simulink model "Vehicle_Dynamics_Test_Simulink"  (R2019a)
settings: Solver=FixedStepAuto  StartTime=0.0  StopTime=300  FixedStep=0.01  RelTol=1e-3
values from neighbouring files (symbols this model uses):
  Braking = Simulink.Parameter    [Vehicle_Dynamics_Script.m]
  Pedalling_Force = Simulink.Parameter    [Vehicle_Dynamics_Script.m]
  Steering_Angle = Simulink.Parameter    [Vehicle_Dynamics_Script.m]
  Terrain = Simulink.Parameter    [Vehicle_Dynamics_Script.m]
libraries: fl_lib x9, nesl_utility x6, sdl_lib x5, simulink_extras x1, vehdynlibsteering x1, autolibshared x1
settings Model: Creator=India  LastModifiedBy=India
settings OptimizationCC: DefaultParameterBehavior=Inlined  EnhancedBackFolding=on  PassReuseOutputArgsAs=Individual arguments  OptimizeBlockOrder=speed  DifferentSizesBufferReuse=on  OptimizationCustomize=off
settings DebuggingCC: ParameterTunabilityLossMsg=error
settings SFSimCC: MATLABDynamicMemAlloc=off
settings RTWCC: SystemTargetFile=ert.tlc  TemplateMakefile=ert_default_tmf  GenerateReport=on  IncludeHyperlinkInReport=on  LaunchReport=on  GenerateTraceInfo=on  GenerateTraceReport=on  GenerateTraceReportSl=on  GenerateTraceReportSf=on  GenerateTraceReportEml=on
settings CodeAppCC: ForceParamTrailComments=on  IgnoreCustomStorageClasses=off  OperatorAnnotations=on  SimulinkDataObjDesc=on  SFDataObjDesc=on  InsertBlockDesc=on
settings ERTTargetCC: TargetLangStandard=C99 (ISO)  GenerateSampleERTMain=on  InlinedParameterPlacement=NonHierarchical  ERTCustomFileTemplate=example_file_process.tlc
settings ConfigComp: DVTestSuiteOptimization=Auto  DVDetectOutOfBounds=on  DVRebuildModelRepresentation=Always

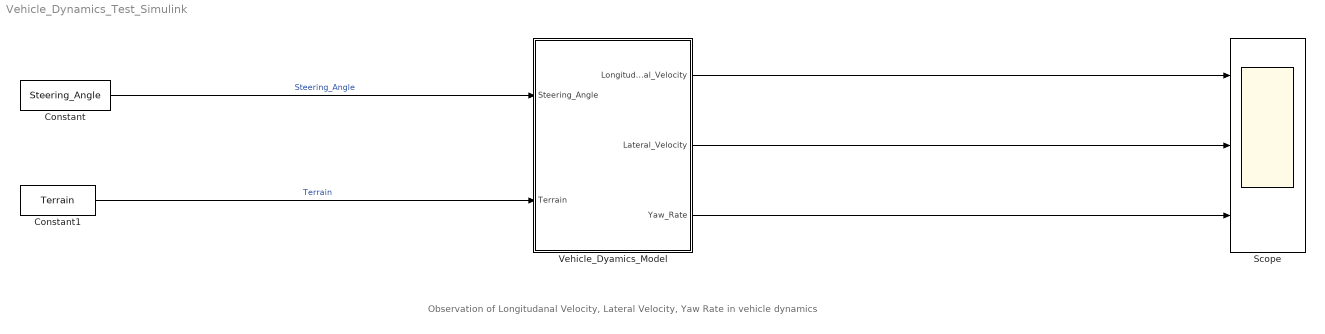
== system Vehicle_Dynamics_Test_Simulink ==
  note: Observation of Longitudanal Velocity, Lateral Velocity, Yaw Rate in vehicle dynamics
  Constant : Constant  Value=Steering_Angle  OutDataTypeStr=double
  Constant1 : Constant  Value=Terrain  OutDataTypeStr=double
  Scope : Scope  NumInputPorts=3
  Vehicle_Dyamics_Model : Subsystem  TreatAsAtomicUnit=on
  wires:
  Constant1/1 -> Vehicle_Dyamics_Model/2(Terrain)  "Terrain"
  Vehicle_Dyamics_Model/2(Lateral_Velocity) -> Scope/2
  Vehicle_Dyamics_Model/3(Yaw_Rate) -> Scope/3
  Constant/1 -> Vehicle_Dyamics_Model/1(Steering_Angle)  "Steering_Angle"
  Vehicle_Dyamics_Model/1(Longitudanal_Velocity) -> Scope/1

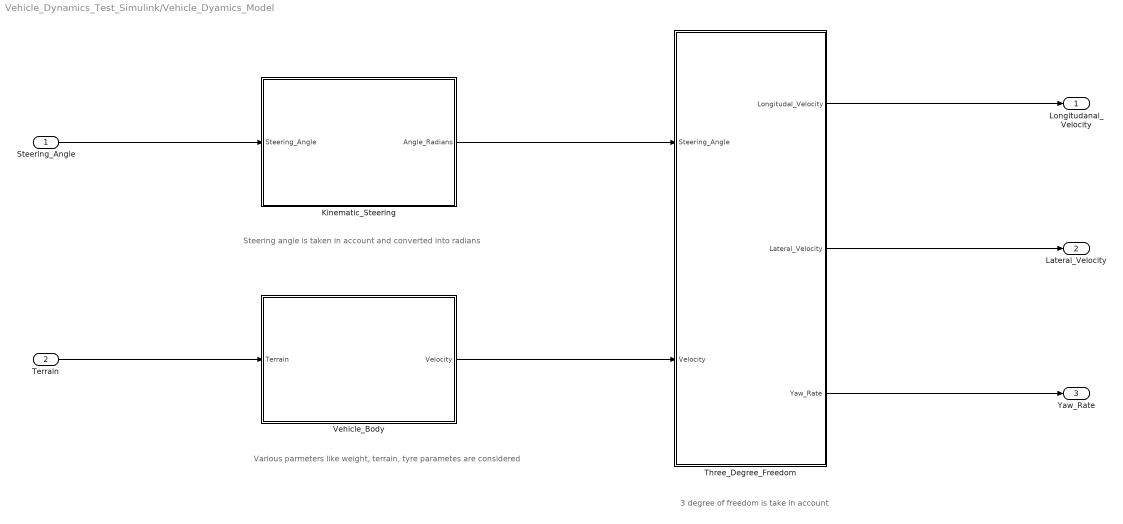
== system Vehicle_Dynamics_Test_Simulink/Vehicle_Dyamics_Model ==
  note: 3 degree of freedom is take in account
  note: Various parmeters like weight, terrain, tyre parametes are considered
  note: Steering angle is taken in account and converted into radians
  Steering_Angle : Inport
  Terrain : Inport  Port=2  OutDataTypeStr=double
  Kinematic_Steering : Subsystem
  Three_Degree_Freedom : Subsystem
  Vehicle_Body : Subsystem
  Longitudanal_Velocity : Outport
  Lateral_Velocity : Outport  Port=2
  Yaw_Rate : Outport  Port=3
  wires:
  Three_Degree_Freedom/1(Longitudal_Velocity) -> Longitudanal_Velocity/1
  Three_Degree_Freedom/2(Lateral_Velocity) -> Lateral_Velocity/1
  Vehicle_Body/1(Velocity) -> Three_Degree_Freedom/2(Velocity)
  Three_Degree_Freedom/3(Yaw_Rate) -> Yaw_Rate/1
  Kinematic_Steering/1(Angle_Radians) -> Three_Degree_Freedom/1(Steering_Angle)
  Terrain/1 -> Vehicle_Body/1(Terrain)
  Steering_Angle/1 -> Kinematic_Steering/1(Steering_Angle)

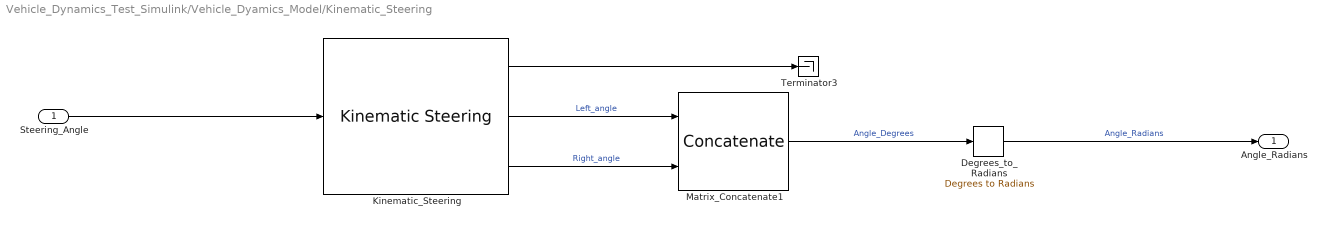
== system Vehicle_Dynamics_Test_Simulink/Vehicle_Dyamics_Model/Kinematic_Steering ==
  Steering_Angle : Inport
  Degrees_to_Radians : simulink_extras/Transformations/Degrees to Radians
  Kinematic_Steering : vehdynlibsteering/Kinematic Steering  StrgType=Ackerman  StrgRatioType=Constant  Loc=Front  NrmlFctr=0.01  TrckWdth=1  WhlBase=1.524  Db=0  StrgRng=1.25*pi  StrgAngBpts="[-6.2832   -5.0265   -3.7699   -2.5133   -1.2566         0    1.2566    2.5133    3.7699    5.0265    6.2832]"  StrgRatioTbl=|  StrgRatio=100  StrgArmLngth=0.1  RckCsLngth=0.5  TieRodLngth=0.248  D=0.2  PnnRadius=0.0057  PnnRadiusTbl="[0.0055    0.0055    0.0056    0.0057    0.0058    0.0057    0.0057    0.0057    0.0056    0.0055    0.0055]"  RodLngth=0.1  ParaArmLngth=0.9  aMode=2
      | [13.5000   13.3750   13.2500   13.1250   13.0000   13.0000   13.0000   13.1250   13.2500   13.3750   13.5000
      | ]
      settings: SourceProductName=Vehicle Dynamics Blockset
  Matrix_Concatenate1 : Concatenate  ConcatenateDimension=2
      settings: AttributesFormatString=%<ConcatenateDimension>
  Terminator3 : Terminator
  Angle_Radians : Outport
  wires:
  Kinematic_Steering/1 -> Terminator3/1
  Kinematic_Steering/3 -> Matrix_Concatenate1/2  "Right_angle"
  Matrix_Concatenate1/1 -> Degrees_to_Radians/1  "Angle_Degrees"
  Kinematic_Steering/2 -> Matrix_Concatenate1/1  "Left_angle"
  Steering_Angle/1 -> Kinematic_Steering/1
  Degrees_to_Radians/1 -> Angle_Radians/1  "Angle_Radians"

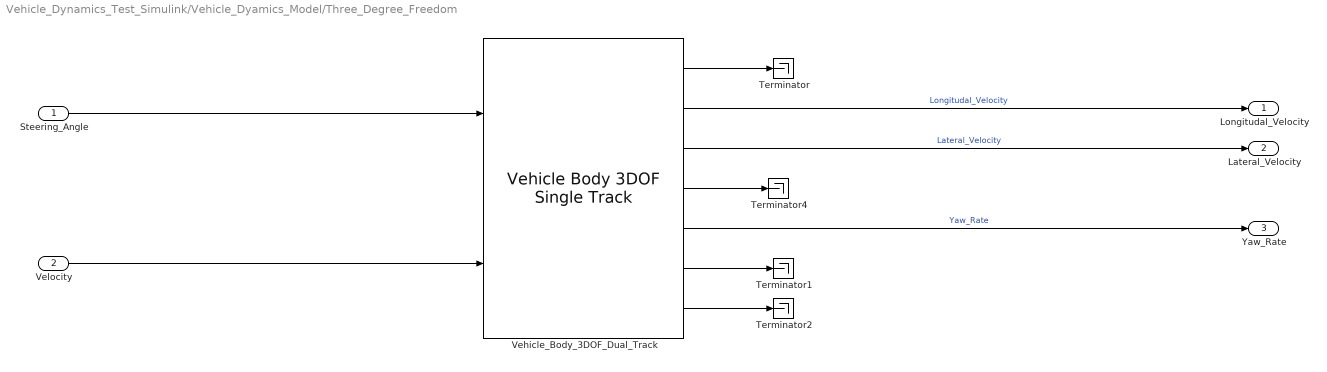
== system Vehicle_Dynamics_Test_Simulink/Vehicle_Dyamics_Model/Three_Degree_Freedom ==
  Steering_Angle : Inport
  Velocity : Inport  Port=2
  Terminator{,1..2,4} (4 alike) : Terminator
  Vehicle_Body_3DOF_Dual_Track : autolibshared/Vehicle Body 3DOF Single Track  trackMode=Dual  inputMode=External longitudinal velocity  frontSteerMode=on  rearSteerMode=off  windMode=off  muMode=off  extFMode=off  extMMode=off  extXo=off  extpsio=off  extxdoto=off  extro=off  extYo=off  extTamb=off  extydoto=off  aMode=2  NF=2  NR=2  m=2000  a=1.4  b=1.6  h=0.35  X_o=0  xdot_o=0  CalphaMode=off  sigmaMode=on  d=0  w=[1.4,1.4]  Cy_f=12e3  Cy_r=11e3  sigma_f=.1  sigma_r=.1  alpha_f_brk=[-.1 .1]  Cy_f_data=[-9e3 9e3]  alpha_r_brk=[-.1 .1]  Cy_r_data=[-9e3 9e3]  Y_o=0  ydot_o=0  Izz=4000  psi_o=0  r_o=0  Af=2  Cd=.3  Cl=.1  Cpm=.1  beta_w=[0:0.01:0.3]  Cs=[0:0.03:0.9]  Cym=[0:0.01:0.3]  Pabs=101325  Tair=273  g=9.81  mu=1  xdot_tol=.01  Fznom=5000  Fxtire_sat=7e4  Fytire_sat=7e4  longOff=0  latOff=0  vertOff=0  wrapAng=off
      settings: SourceProductName=Powertrain Blockset  SourceProductBaseCode=PW
  Longitudal_Velocity : Outport
  Lateral_Velocity : Outport  Port=2
  Yaw_Rate : Outport  Port=3
  wires:
  Vehicle_Body_3DOF_Dual_Track/3 -> Lateral_Velocity/1  "Lateral_Velocity"
  Vehicle_Body_3DOF_Dual_Track/6 -> Terminator1/1
  Velocity/1 -> Vehicle_Body_3DOF_Dual_Track/2
  Vehicle_Body_3DOF_Dual_Track/7 -> Terminator2/1
  Vehicle_Body_3DOF_Dual_Track/1 -> Terminator/1
  Vehicle_Body_3DOF_Dual_Track/4 -> Terminator4/1
  Vehicle_Body_3DOF_Dual_Track/5 -> Yaw_Rate/1  "Yaw_Rate"
  Steering_Angle/1 -> Vehicle_Body_3DOF_Dual_Track/1
  Vehicle_Body_3DOF_Dual_Track/2 -> Longitudal_Velocity/1  "Longitudal_Velocity"

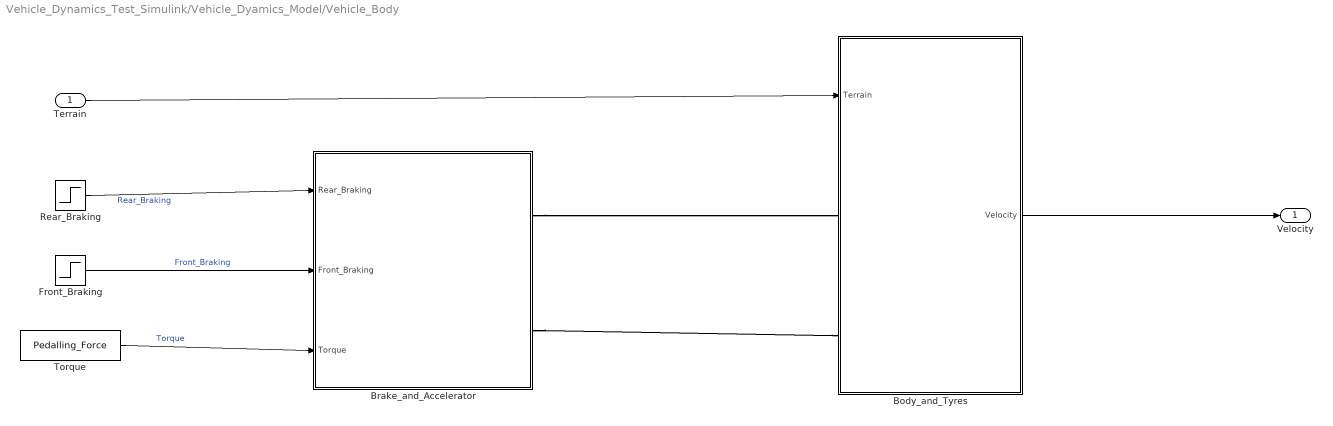
== system Vehicle_Dynamics_Test_Simulink/Vehicle_Dyamics_Model/Vehicle_Body ==
  Terrain : Inport  OutDataTypeStr=double
  Body_and_Tyres : Subsystem
  Brake_and_Accelerator : Subsystem
  Front_Braking : Step  Time=100  After=Terrain  SampleTime=0
  Rear_Braking : Step  Time=100  After=Braking  SampleTime=0
  Torque : Constant  Value=Pedalling_Force
  Velocity : Outport
  wires:
  Rear_Braking/1 -> Brake_and_Accelerator/1(Rear_Braking)  "Rear_Braking"
  Front_Braking/1 -> Brake_and_Accelerator/2(Front_Braking)  "Front_Braking"
  Torque/1 -> Brake_and_Accelerator/3(Torque)  "Torque"
  Terrain/1 -> Body_and_Tyres/1(Terrain)
  Body_and_Tyres/1(Velocity) -> Velocity/1
  connections:
  Brake_and_Accelerator/RConn1 -- Body_and_Tyres/LConn1
  Brake_and_Accelerator/RConn2 -- Body_and_Tyres/LConn2

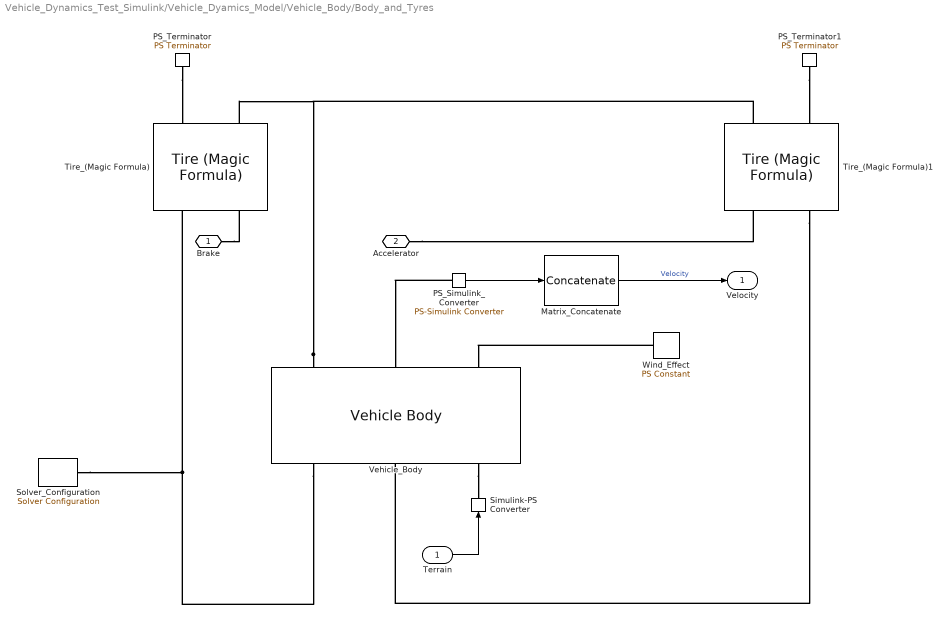
== system Vehicle_Dynamics_Test_Simulink/Vehicle_Dyamics_Model/Vehicle_Body/Body_and_Tyres ==
  Terrain : Inport
  Matrix_Concatenate : Concatenate  NumInputs=1  ConcatenateDimension=2
      settings: AttributesFormatString=%<ConcatenateDimension>
  PS_Simulink_Converter : nesl_utility/PS-Simulink Converter  PhysicalDomain=network_engine_domain  SubClassName=ps_output  LeftPortType=input  RightPortType=output  PseudoPeriodic=off  Frequencies=[]  Unit=1  AffineConversion=off
  PS_Terminator : fl_lib/Physical Signals/Sinks/PS Terminator
      settings: SourceProductName=Simscape
  PS_Terminator1 : fl_lib/Physical Signals/Sinks/PS Terminator
      settings: SourceProductName=Simscape
  Simulink-PS Converter : nesl_utility/Simulink-PS Converter  PhysicalDomain=network_engine_domain  SubClassName=ps_input  LeftPortType=input  RightPortType=output  PseudoPeriodic=off  Frequencies=[]  NoiseDistribution=none  NoiseParameters=[]  Unit=1  AffineConversion=off  FilteringAndDerivatives=provide  SimscapeFilterOrder=1  InputFilterTimeConstant=0.001  UdotUserProvided=0
  Solver_Configuration : nesl_utility/Solver Configuration  PhysicalDomain=network_engine_domain  SubClassName=solver  LeftPortType=input  RightPortType=generic  Tones=[]  Harmonics=[]  SimulateNoise=off  Profile=off  UseLocalSampling=off  EnableSwitchedLinearOptims=on  FrequencyDomain=off  UseCCode=off  RelTol=0.001  AbsTol=1e-06  MinStep=1e-09  ToWorkspace=off  RevertToSquareIcSolve=off  NumHomotopyIterations=100  PhasorMode=off  PhasorModeNumHarmonics=1  DoDC=off  ResidualTolerance=1e-09  UseLocalSolver=off  LocalSolverChoice=NE_BACKWARD_EULER_ADVANCER  LocalSolverSampleTime=0.001  DoFixedCost=off  MaxNonlinIter=3  MaxModeIter=2  LinearAlgebra=auto  EquationFormulation=NE_TIME_EF  DelaysMemoryBudget=1024  AutomaticFiltering=on  FilteringTimeConstant=0.001  PartitionStorageMethod=AS_NEEDED  PartitionMemoryBudget=1024  PartitionMethod=ROBUST
  Tire_(Magic Formula) : sdl_lib/Tires & Vehicles/Tire (Magic Formula)  parameterization=sdl.enum.magic_tire_model.constant  F_z1=3000 N  F_x1=3500 N  kappa1=10  B_m=10  C_m=1.9  D_m=1  E_m=0.97  fz0=4000 N  p_Cx=1.685  p_Dx=[1.21, -.037]  p_Ex=[.344, .095, -.02, 0]  p_Kx=[21.51, -.163, .245]  p_Hx=[-.002, .002]  p_Vx=[0, 0]  v_tr_thr=0.1 m/s  r_e=0.45 m  model_compliance=0  stiffness=1e6 N/m  damping=1000 N/(m/s)  model_inertia=1  inertia=1e-3 kg*m^2  initial_velocity=0 rad/s  model_resistance=1  resistance_model=1  coeff=0.005  p_tire=250e3 Pa  alpha=-0.003  beta=0.97  coeff_a=84e-4  coeff_b=6.2e-4 s/m  coeff_c=1.6e-4 s^2/m^2  v_thr=0.001 m/s
      settings: SourceProductName=Simscape Driveline
  Tire_(Magic Formula)1 : sdl_lib/Tires & Vehicles/Tire (Magic Formula)  parameterization=sdl.enum.magic_tire_model.constant  F_z1=3000 N  F_x1=3500 N  kappa1=10  B_m=10  C_m=1.9  D_m=1  E_m=0.97  fz0=4000 N  p_Cx=1.685  p_Dx=[1.21, -.037]  p_Ex=[.344, .095, -.02, 0]  p_Kx=[21.51, -.163, .245]  p_Hx=[-.002, .002]  p_Vx=[0, 0]  v_tr_thr=0.1 m/s  r_e=0.45 m  model_compliance=0  stiffness=1e6 N/m  damping=1000 N/(m/s)  model_inertia=1  inertia=1e-3 kg*m^2  initial_velocity=0 rad/s  model_resistance=1  resistance_model=1  coeff=0.005  p_tire=250e3 Pa  alpha=-0.003  beta=0.97  coeff_a=84e-4  coeff_b=6.2e-4 s/m  coeff_c=1.6e-4 s^2/m^2  v_thr=0.001 m/s
      settings: SourceProductName=Simscape Driveline
  Vehicle_Body : sdl_lib/Tires & Vehicles/Vehicle Body  mass=1400 kg  n_w=2  x_f=0.95 m  x_r=0.95 m  y_c=0.95 m  mass_var=simscape.enum.onoff.off  model_pitch=simscape.enum.onoff.on  inertia=1263.5 kg*m^2  suspension_model=sdl.enum.linearTLU.linear  k_f=18000 N/m  b_f=1500 N/(m/s)  k_r=18000 N/m  b_r=1500 N/(m/s)  k_f_TLU=[-2000, -1000, 0, 1000, 2000] N  x_f_TLU=[-.4, -.2, 0, .2, .4] m  b_f_TLU=[-200, -100, 0, 100, 200] N  v_f_TLU=[-4, -2, 0, 2, 4] m/s  k_r_TLU=[-2000, -1000, 0, 1000, 2000] N  x_r_TLU=[-.4, -.2, 0, .2, .4] m  b_r_TLU=[-200, -100, 0, 100, 200] N  v_r_TLU=[-4, -2, 0, 2, 4] m/s  interp_method=simscape.enum.interpolation.linear  extrap_method=simscape.enum.extrapolation.linear  model_hardstop=simscape.enum.onoff.off  upper_bound_f=.25 m  lower_bound_f=-.25 m  stop_k_f=1e6 N/m  stop_b_f=150 N/(m/s)  upper_bound_r=.25 m  lower_bound_r=-.25 m  stop_k_r=1e6 N/m  stop_b_r=150 N/(m/s)  initial_pitch=0 rad  initial_pitch_rate=0 rad/s  g=9.81 m/s^2  liftoff_warning=simscape.enum.onoff.off  area=1.33 m^2  Cd=1.2  rho=1.2 kg/m^3  v_specify=off  v_priority=High  v=0 m/s  v_nominal_specify=off  v_nominal_unit=m/s  v_nominal_value=1
      settings: SourceProductName=Simscape Driveline
  Wind_Effect : fl_lib/Physical Signals/Sources/PS Constant  constant=1
  Brake : PMIOPort  Side=Left
  Accelerator : PMIOPort  Port=2  Side=Left
  Velocity : Outport
  wires:
  PS_Simulink_Converter/1 -> Matrix_Concatenate/1
  Matrix_Concatenate/1 -> Velocity/1  "Velocity"
  Terrain/1 -> Simulink-PS Converter/1
  connections:
  Vehicle_Body/LConn1 -- Tire_(Magic Formula)/RConn2 -- Tire_(Magic Formula)1/RConn2
  PS_Simulink_Converter/LConn1 -- Vehicle_Body/LConn2
  Vehicle_Body/RConn1 -- Solver_Configuration/RConn1 -- Tire_(Magic Formula)/LConn1
  PS_Terminator/LConn1 -- Tire_(Magic Formula)/RConn1
  PS_Terminator1/LConn1 -- Tire_(Magic Formula)1/RConn1
  Vehicle_Body/RConn3 -- Simulink-PS Converter/RConn1
  Tire_(Magic Formula)1/LConn1 -- Vehicle_Body/RConn2
  Brake/RConn1 -- Tire_(Magic Formula)/LConn2
  Wind_Effect/RConn1 -- Vehicle_Body/LConn3
  Accelerator/RConn1 -- Tire_(Magic Formula)1/LConn2

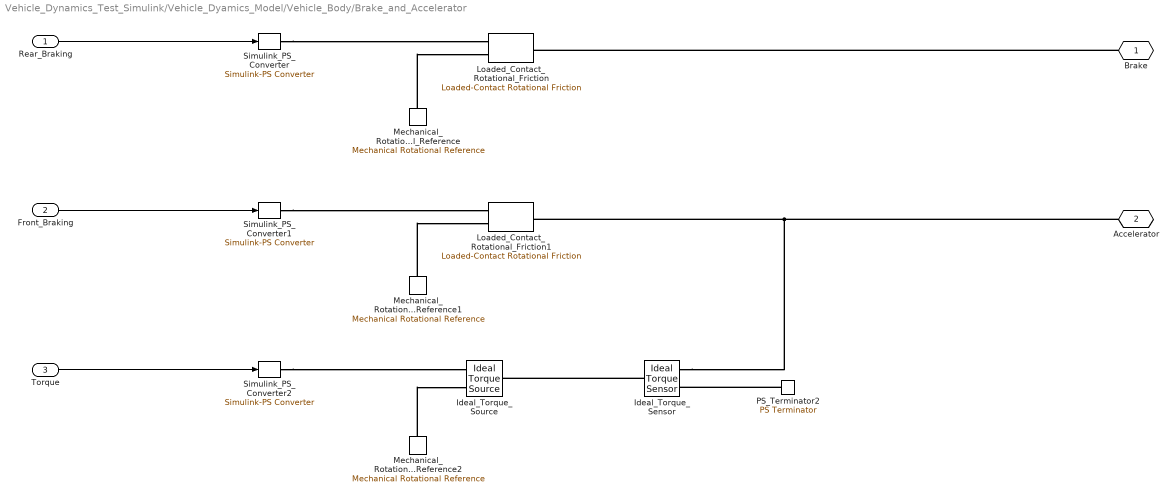
== system Vehicle_Dynamics_Test_Simulink/Vehicle_Dyamics_Model/Vehicle_Body/Brake_and_Accelerator ==
  Rear_Braking : Inport
  Front_Braking : Inport  Port=2
  Torque : Inport  Port=3
  Ideal_Torque_Sensor : fl_lib/Mechanical/Mechanical Sensors/Ideal Torque Sensor
  Ideal_Torque_Source : fl_lib/Mechanical/Mechanical Sources/Ideal Torque Source
  Loaded_Contact_Rotational_Friction : sdl_lib/Brakes & Detents/Rotational/Loaded-Contact Rotational Friction  geometry_model=1  r_eff=130 mm  d_o=150 mm  d_i=100 mm  friction_model=1  mu_coulomb=0.3  mu_w_vector=[0, 100, 1000] rad/s  mu_coulomb_vector=[.3, .22, .19]  mu_interp_method=simscape.enum.interpolation.linear  mu_extrap_method=simscape.enum.extrapolation.linear  mu_static=0.35  w_tol=0.001 rad/s  force_min=1 N  mu_visc=0 N*m/(rad/s)  initial_state_locked=0  temperature_TLU=[280, 300, 320] K  mu_coulomb_temp_vector=[.3, .28, .25]  mu_coulomb_matrix=[.34, .32, .3; .3, .28, .25; .25, .2, .15]  mu_static_vector=[.4, .38, .36]  thermal_mass=50 kJ/K  T_init=300 K
      settings: SourceProductName=Simscape Driveline  SourceProductBaseCode=LD
  Loaded_Contact_Rotational_Friction1 : sdl_lib/Brakes & Detents/Rotational/Loaded-Contact Rotational Friction  geometry_model=1  r_eff=130 mm  d_o=150 mm  d_i=100 mm  friction_model=1  mu_coulomb=0.3  mu_w_vector=[0, 100, 1000] rad/s  mu_coulomb_vector=[.3, .22, .19]  mu_interp_method=simscape.enum.interpolation.linear  mu_extrap_method=simscape.enum.extrapolation.linear  mu_static=0.35  w_tol=0.001 rad/s  force_min=1 N  mu_visc=0 N*m/(rad/s)  initial_state_locked=0  temperature_TLU=[280, 300, 320] K  mu_coulomb_temp_vector=[.3, .28, .25]  mu_coulomb_matrix=[.34, .32, .3; .3, .28, .25; .25, .2, .15]  mu_static_vector=[.4, .38, .36]  thermal_mass=50 kJ/K  T_init=300 K
      settings: SourceProductName=Simscape Driveline  SourceProductBaseCode=LD
  Mechanical_Rotational_Reference : fl_lib/Mechanical/Rotational Elements/Mechanical Rotational Reference
  Mechanical_Rotational_Reference1 : fl_lib/Mechanical/Rotational Elements/Mechanical Rotational Reference
  Mechanical_Rotational_Reference2 : fl_lib/Mechanical/Rotational Elements/Mechanical Rotational Reference
  PS_Terminator2 : fl_lib/Physical Signals/Sinks/PS Terminator
      settings: SourceProductName=Simscape
  Simulink_PS_Converter : nesl_utility/Simulink-PS Converter  PhysicalDomain=network_engine_domain  SubClassName=ps_input  LeftPortType=input  RightPortType=output  PseudoPeriodic=off  Frequencies=[]  NoiseDistribution=none  NoiseParameters=[]  Unit=1  AffineConversion=off  FilteringAndDerivatives=provide  SimscapeFilterOrder=1  InputFilterTimeConstant=0.001  UdotUserProvided=0
  Simulink_PS_Converter1 : nesl_utility/Simulink-PS Converter  PhysicalDomain=network_engine_domain  SubClassName=ps_input  LeftPortType=input  RightPortType=output  PseudoPeriodic=off  Frequencies=[]  NoiseDistribution=none  NoiseParameters=[]  Unit=1  AffineConversion=off  FilteringAndDerivatives=provide  SimscapeFilterOrder=1  InputFilterTimeConstant=0.001  UdotUserProvided=0
  Simulink_PS_Converter2 : nesl_utility/Simulink-PS Converter  PhysicalDomain=network_engine_domain  SubClassName=ps_input  LeftPortType=input  RightPortType=output  PseudoPeriodic=off  Frequencies=[]  NoiseDistribution=none  NoiseParameters=[]  Unit=1  AffineConversion=off  FilteringAndDerivatives=provide  SimscapeFilterOrder=1  InputFilterTimeConstant=0.001  UdotUserProvided=0
  Brake : PMIOPort  Side=Right
  Accelerator : PMIOPort  Port=2  Side=Right
  wires:
  Front_Braking/1 -> Simulink_PS_Converter1/1
  Torque/1 -> Simulink_PS_Converter2/1
  Rear_Braking/1 -> Simulink_PS_Converter/1
  connections:
  Ideal_Torque_Sensor/LConn1 -- Ideal_Torque_Source/LConn1
  Simulink_PS_Converter2/RConn1 -- Ideal_Torque_Source/RConn1
  Mechanical_Rotational_Reference/LConn1 -- Loaded_Contact_Rotational_Friction/LConn2
  Simulink_PS_Converter1/RConn1 -- Loaded_Contact_Rotational_Friction1/LConn1
  Simulink_PS_Converter/RConn1 -- Loaded_Contact_Rotational_Friction/LConn1
  PS_Terminator2/LConn1 -- Ideal_Torque_Sensor/RConn2
  Mechanical_Rotational_Reference2/LConn1 -- Ideal_Torque_Source/RConn2
  Mechanical_Rotational_Reference1/LConn1 -- Loaded_Contact_Rotational_Friction1/LConn2
  Brake/RConn1 -- Loaded_Contact_Rotational_Friction/RConn1
  Accelerator/RConn1 -- Ideal_Torque_Sensor/RConn1 -- Loaded_Contact_Rotational_Friction1/RConn1
